simulink model "HCU_V2_Simulink"  (R2025b)
settings: Solver=FixedStepDiscrete  StartTime=0.0  StopTime=10.0  FixedStep=0.01  RelTol=1e-3
libraries: simulink x30, hdlsllib x9, etargetslib x7
(part 1 of 2)
settings Model: Creator=Yusha  LastModifiedBy=Yusha
settings OptimizationCC: DefaultParameterBehavior=Inlined  EnhancedBackFolding=on  PassReuseOutputArgsAs=Individual arguments  ZeroExternalMemoryAtStartup=off  ZeroInternalMemoryAtStartup=off  OptimizeBlockOrder=speed  DifferentSizesBufferReuse=on  OptimizationCustomize=off  EfficientTunableParamExpr=on
settings DebuggingCC: ParameterTunabilityLossMsg=error
settings HardwareCC: ProdBitPerPointer=32.0  ProdBitPerSizeT=32.0  ProdBitPerPtrDiffT=32.0  ProdLargestAtomicInteger=Long  ProdLargestAtomicFloat=Double  ProdWordSize=32.0  ProdHWDeviceType=ARM Compatible->ARM Cortex-M
settings SFSimCC: MATLABDynamicMemAlloc=off
settings RTWCC: SystemTargetFile=ert.tlc  GenCodeOnly=on  TemplateMakefile=ert_default_tmf  Description=Embedded Coder
settings CodeAppCC: ForceParamTrailComments=on  IgnoreCustomStorageClasses=off  OperatorAnnotations=on  SimulinkDataObjDesc=on  SFDataObjDesc=on  InsertBlockDesc=on
settings ERTTargetCC: ERTCustomFileTemplate=example_file_process.tlc  TargetLangStandard=C99 (ISO)

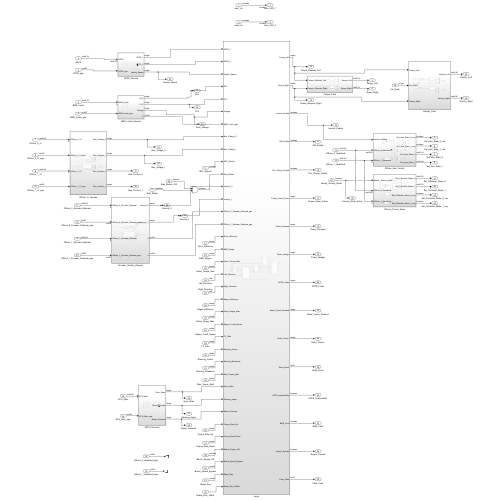
[thumbnail: Simulink's stored preview of the top-level diagram]
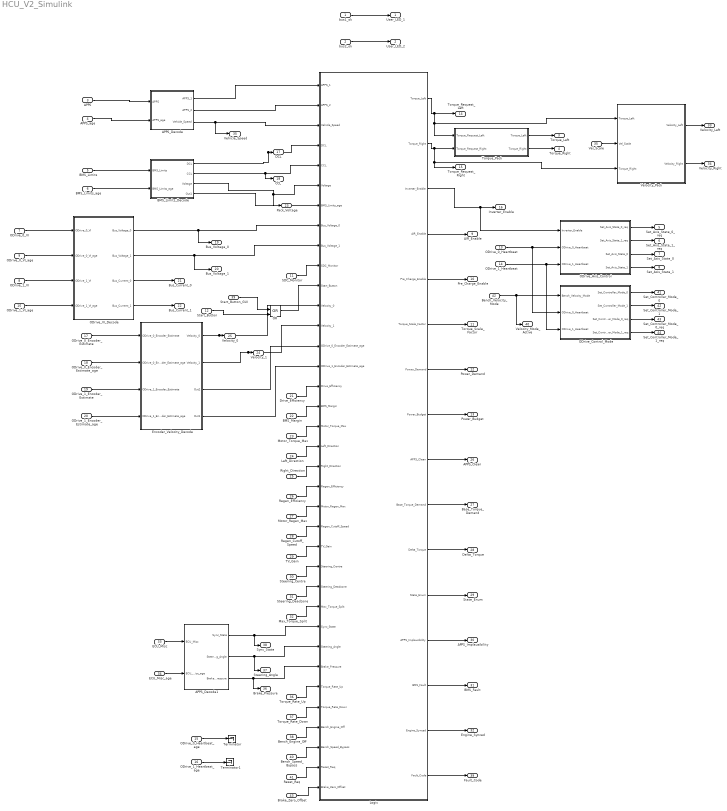
== system HCU_V2_Simulink ==
  bus1_ok : Inport  OutDataTypeStr=boolean
  bus2_ok : Inport  Port=2  OutDataTypeStr=boolean
  APPS : Inport  Port=3
  APPS_age : Inport  Port=4  OutDataTypeStr=uint32
  BMS_Limits : Inport  Port=5  OutDataTypeStr=uint8
  BMS_Limits_age : Inport  Port=6  OutDataTypeStr=uint32
  ODrive_0_VI : Inport  Port=7  OutDataTypeStr=uint8  PortDimensions=8
  ODrive_1_VI : Inport  Port=8  OutDataTypeStr=uint8  PortDimensions=8
  ODrive_0_VI_age : Inport  Port=9  OutDataTypeStr=uint32
  ODrive_1_VI_age : Inport  Port=10  OutDataTypeStr=uint32
  SDC_Monitor : Inport  Port=11  OutDataTypeStr=boolean
  Start_Button : Inport  Port=12  OutDataTypeStr=boolean
  ODrive_0_Heartbeat : Inport  Port=13  OutDataTypeStr=uint8  PortDimensions=8
  ODrive_1_Heartbeat : Inport  Port=14
  ODrive_0_Heartbeat_age : Inport  Port=15  OutDataTypeStr=uint32
  ODrive_1_Heartbeat_age : Inport  Port=16  OutDataTypeStr=uint32
  ODrive_0_Encoder_Estimate : Inport  Port=17  OutDataTypeStr=uint8  PortDimensions=8
  ODrive_0_Encoder_Estimate_age : Inport  Port=18  OutDataTypeStr=uint32
  ODrive_1_Encoder_Estimate : Inport  Port=19  OutDataTypeStr=uint8  PortDimensions=8
  ODrive_1_Encoder_Estimate_age : Inport  Port=20  OutDataTypeStr=uint32
  Drive_Efficiency : Inport  Port=21  OutDataTypeStr=single
  BMS_Margin : Inport  Port=22  OutDataTypeStr=single
  Motor_Torque_Max : Inport  Port=23  OutDataTypeStr=single
  Left_Direction : Inport  Port=24  OutDataTypeStr=int8
  Right_Direction : Inport  Port=25  OutDataTypeStr=int8
  Regen_Efficiency : Inport  Port=26  OutDataTypeStr=single
  Motor_Regen_Max : Inport  Port=27  OutDataTypeStr=single
  Regen_Cutoff_Speed : Inport  Port=28  OutDataTypeStr=single
  TV_Gain : Inport  Port=29
  Steering_Centre : Inport  Port=30
  Steering_Deadzone : Inport  Port=31
  Max_Torque_Split : Inport  Port=32
  ECU_Misc : Inport  Port=33  OutDataTypeStr=uint8  PortDimensions=8
  ECU_Misc_age : Inport  Port=34  OutDataTypeStr=uint32
  Vel_Scale : Inport  Port=35  OutDataTypeStr=single
  Torque_Rate_Up : Inport  Port=36
  Torque_Rate_Down : Inport  Port=37
  Bench_Engine_Off : Inport  Port=38  OutDataTypeStr=boolean
  Start_Button_GUI : Inport  Port=39
  Bench_Speed_Bypass : Inport  Port=40
  Reset_Req : Inport  Port=41
  Bench_Velocity_Mode : Inport  Port=42  OutDataTypeStr=boolean
  Brake_Zero_Offset : Inport  Port=43
  APPS_Decode : Subsystem
  APPS_Decode1 : Subsystem
  BMS_Limits_Decode : Subsystem
  Encoder_Velocity_Decode : Subsystem
  Logic : Subsystem
  ODrive_Axis_Control : Subsystem
  ODrive_Control_Mode : Subsystem
  ODrive_VI_Decode : Subsystem
  OR : Logic  Operator=OR  IconShape=distinctive  AllPortsSameDT=off  OutDataTypeStr=boolean
  Terminator : Terminator
  Terminator1 : Terminator
  Torque_Pack : Subsystem
  Velocity_Pack : Subsystem
  User_LED_1 : Outport  OutDataTypeStr=boolean
  User_LED_2 : Outport  Port=2  OutDataTypeStr=boolean
  Torque_Left : Outport  Port=3
  Torque_Right : Outport  Port=4
  Set_Axis_State_0_req : Outport  Port=5
  Set_Axis_State_1_req : Outport  Port=6
  Set_Axis_State_0 : Outport  Port=7
  Set_Axis_State_1 : Outport  Port=8
  AIR_Enable : Outport  Port=9
  Pre_Charge_Enable : Outport  Port=10
  Torque_Scale_Factor : Outport  Port=11
  Power_Demand : Outport  Port=12
  Power_Budget : Outport  Port=13
  Torque_Request_Left : Outport  Port=14
  Torque_Request_Right : Outport  Port=15
  Inverter_Enable : Outport  Port=16
  DCL : Outport  Port=17
  CCL : Outport  Port=18
  Bus_Voltage_0 : Outport  Port=19
  Bus_Voltage_1 : Outport  Port=20
  Bus_Current_0 : Outport  Port=21
  Bus_Current_1 : Outport  Port=22
  Pack_Voltage : Outport  Port=23
  Velocity_1 : Outport  Port=24
  Velocity_0 : Outport  Port=25
  APPS_Clean : Outport  Port=26
  Base_Torque_Demand : Outport  Port=27
  "Delta_Torque " : Outport  Port=28
  State_Enum : Outport  Port=29
  APPS_Implausibility : Outport  Port=30
  BMS_Fault : Outport  Port=31
  Engine_Synced : Outport  Port=32
  Velocity_Left : Outport  Port=33
  Velocity_Right : Outport  Port=34
  Vehicle_Speed : Outport  Port=35
  Brake_Pressure : Outport  Port=36
  Steering_Angle : Outport  Port=37
  Sync_State : Outport  Port=38
  Fault_Code : Outport  Port=39
  Velocity_Mode_Active : Outport  Port=40
  Set_Controller_Mode_0 : Outport  Port=41
  Set_Controller_Mode_1 : Outport  Port=42
  Set_Controller_Mode_0_req : Outport  Port=43
  Set_Controller_Mode_1_req : Outport  Port=44
  wires:
  bus2_ok/1 -> User_LED_2/1
  bus1_ok/1 -> User_LED_1/1
  APPS/1 -> APPS_Decode/1(APPS)
  APPS_age/1 -> APPS_Decode/2(APPS_age)
  APPS_Decode/1(APPS_1) -> Logic/1(APPS_1)
  APPS_Decode/2(APPS_2) -> Logic/2(APPS_2)
  BMS_Limits/1 -> BMS_Limits_Decode/1(BMS_Limits)
  BMS_Limits_age/1 -> BMS_Limits_Decode/2(BMS_Limits_age)
  BMS_Limits_Decode/1(DCL) -> DCL/1, Logic/4(DCL)
  BMS_Limits_Decode/2(CCL) -> CCL/1, Logic/5(CCL)
  BMS_Limits_Decode/3(Voltage) -> Pack_Voltage/1, Logic/6(Voltage)
  ODrive_0_VI/1 -> ODrive_VI_Decode/1(ODrive_0_VI)
  ODrive_0_VI_age/1 -> ODrive_VI_Decode/2(ODrive_0_VI_age)
  ODrive_1_VI/1 -> ODrive_VI_Decode/3(ODrive_1_VI)
  ODrive_1_VI_age/1 -> ODrive_VI_Decode/4(ODrive_1_VI_age)
  ODrive_VI_Decode/1(Bus_Voltage_0) -> Bus_Voltage_0/1, Logic/8(Bus_Voltage_0)
  ODrive_VI_Decode/2(Bus_Voltage_1) -> Bus_Voltage_1/1, Logic/9(Bus_Voltage_1)
  Logic/1(Torque_Left) -> Torque_Pack/1(Torque_Request_Left), Velocity_Pack/1(Torque_Left), Torque_Request_Left/1
  Logic/2(Torque_Right) -> Torque_Request_Right/1, Velocity_Pack/3(Torque_Right), Torque_Pack/2(Torque_Request_Right)
  Torque_Pack/1(Torque_Left) -> Torque_Left/1
  Torque_Pack/2(Torque_Right) -> Torque_Right/1
  Logic/3(Inverter_Enable) -> ODrive_Axis_Control/1(Inverter_Enable), Inverter_Enable/1
  ODrive_0_Heartbeat/1 -> ODrive_Axis_Control/2(ODrive_0_Heartbeat), ODrive_Control_Mode/2(ODrive_0_Heartbeat)
  ODrive_1_Heartbeat/1 -> ODrive_Control_Mode/3(ODrive_1_Heartbeat), ODrive_Axis_Control/3(ODrive_1_Heartbeat)
  ODrive_Axis_Control/1(Set_Axis_State_0_req) -> Set_Axis_State_0_req/1
  ODrive_Axis_Control/2(Set_Axis_State_1_req) -> Set_Axis_State_1_req/1
  ODrive_Axis_Control/3(Set_Axis_State_0) -> Set_Axis_State_0/1
  ODrive_Axis_Control/4(Set_Axis_State_1) -> Set_Axis_State_1/1
  Logic/4(AIR_Enable) -> AIR_Enable/1
  Logic/5(Pre_Charge_Enable) -> Pre_Charge_Enable/1
  ODrive_0_Heartbeat_age/1 -> Terminator/1
  ODrive_1_Heartbeat_age/1 -> Terminator1/1
  ODrive_0_Encoder_Estimate/1 -> Encoder_Velocity_Decode/1(ODrive_0_Encoder_Estimate)
  ODrive_0_Encoder_Estimate_age/1 -> Encoder_Velocity_Decode/2(ODrive_0_Encoder_Estimate_age)
  ODrive_1_Encoder_Estimate/1 -> Encoder_Velocity_Decode/3(ODrive_1_Encoder_Estimate)
  ODrive_1_Encoder_Estimate_age/1 -> Encoder_Velocity_Decode/4(ODrive_1_Encoder_Estimate_age)
  Encoder_Velocity_Decode/1(Velocity_0) -> Logic/12(Velocity_0), Velocity_0/1
  Encoder_Velocity_Decode/2(Velocity_1) -> Velocity_1/1, Logic/13(Velocity_1)
  Encoder_Velocity_Decode/3(Out2) -> Logic/14(ODrive_0_Encoder_Estimate_age)
  Encoder_Velocity_Decode/4(Out1) -> Logic/15(ODrive_1_Encoder_Estimate_age)
  BMS_Limits_Decode/4(Out1) -> Logic/7(BMS_Limits_age)
  Drive_Efficiency/1 -> Logic/16(Drive_Efficiency)
  BMS_Margin/1 -> Logic/17(BMS_Margin)
  Motor_Torque_Max/1 -> Logic/18(Motor_Torque_Max)
  Left_Direction/1 -> Logic/19(Left_Direction)
  Right_Direction/1 -> Logic/20(Right_Direction)
  Logic/6(Torque_Scale_Factor) -> Torque_Scale_Factor/1
  Logic/7(Power_Demand) -> Power_Demand/1
  Logic/8(Power_Budget) -> Power_Budget/1
  Regen_Efficiency/1 -> Logic/21(Regen_Efficiency)
  Motor_Regen_Max/1 -> Logic/22(Motor_Regen_Max)
  Regen_Cutoff_Speed/1 -> Logic/23(Regen_Cutoff_Speed)
  ODrive_VI_Decode/3(Bus_Current_0) -> Bus_Current_0/1
  ODrive_VI_Decode/4(Bus_Current_1) -> Bus_Current_1/1
  Logic/9(APPS_Clean) -> APPS_Clean/1
  Logic/10(Base_Torque_Demand) -> Base_Torque_Demand/1
  TV_Gain/1 -> Logic/24(TV_Gain)
  Steering_Centre/1 -> Logic/25(Steering_Centre)
  Steering_Deadzone/1 -> Logic/26(Steering_Deadzone)
  Max_Torque_Split/1 -> Logic/27(Max_Torque_Split)
  Logic/11("Delta_Torque ") -> "Delta_Torque "/1
  Logic/12(State_Enum) -> State_Enum/1
  Logic/13(APPS_Implausibility) -> APPS_Implausibility/1
  Logic/14(BMS_Fault) -> BMS_Fault/1
  ECU_Misc/1 -> APPS_Decode1/1(ECU_Misc)
  ECU_Misc_age/1 -> APPS_Decode1/2(ECU_Misc_age)
  APPS_Decode1/2(Steering_Angle) -> Steering_Angle/1, Logic/29(Steering_Angle)
  APPS_Decode1/3(Brake_Pressure) -> Brake_Pressure/1, Logic/30(Brake_Pressure)
  APPS_Decode1/1(Sync_State) -> Sync_State/1, Logic/28(Sync_State)
  Logic/15(Engine_Synced) -> Engine_Synced/1
  Vel_Scale/1 -> Velocity_Pack/2(Vel_Scale)
  Velocity_Pack/1(Velocity_Left) -> Velocity_Left/1
  Velocity_Pack/2(Velocity_Right) -> Velocity_Right/1
  Torque_Rate_Up/1 -> Logic/31(Torque_Rate_Up)
  Torque_Rate_Down/1 -> Logic/32(Torque_Rate_Down)
  Bench_Engine_Off/1 -> Logic/33(Bench_Engine_Off)
  OR/1 -> Logic/11(Start_Button)
  SDC_Monitor/1 -> Logic/10(SDC_Monitor)
  Start_Button_GUI/1 -> OR/1
  APPS_Decode/3(Vehicle_Speed) -> Vehicle_Speed/1, Logic/3(Vehicle_Speed)
  Bench_Speed_Bypass/1 -> Logic/34(Bench_Speed_Bypass)
  Start_Button/1 -> OR/2
  Logic/16(Fault_Code) -> Fault_Code/1
  Reset_Req/1 -> Logic/35(Reset_Req)
  Bench_Velocity_Mode/1 -> Velocity_Mode_Active/1, ODrive_Control_Mode/1(Bench_Velocity_Mode)
  ODrive_Control_Mode/1(Set_Controller_Mode_0) -> Set_Controller_Mode_0/1
  ODrive_Control_Mode/2(Set_Controller_Mode_1) -> Set_Controller_Mode_1/1
  ODrive_Control_Mode/3(Set_Controller_Mode_0_req) -> Set_Controller_Mode_0_req/1
  ODrive_Control_Mode/4(Set_Controller_Mode_1_req) -> Set_Controller_Mode_1_req/1
  Brake_Zero_Offset/1 -> Logic/36(Brake_Zero_Offset)

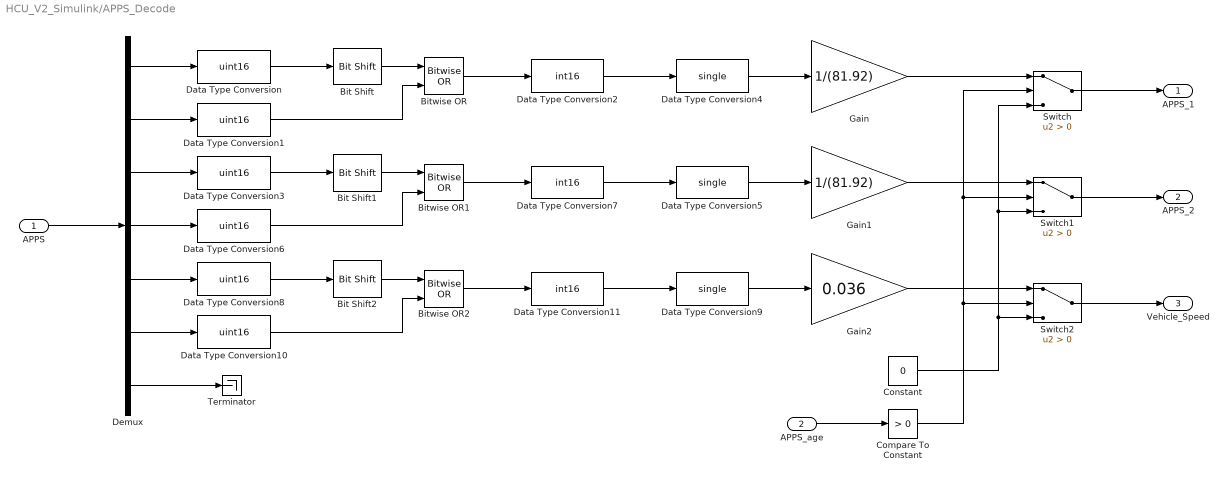
== system HCU_V2_Simulink/APPS_Decode ==
  APPS : Inport  OutDataTypeStr=uint8  PortDimensions=8
  APPS_age : Inport  Port=2
  Bit Shift : hdlsllib/Logic and Bit Operations/Bit Shift  mode=Shift Left Logical  N=8
  Bit Shift1 : hdlsllib/Logic and Bit Operations/Bit Shift  mode=Shift Left Logical  N=8
  Bit Shift2 : hdlsllib/Logic and Bit Operations/Bit Shift  mode=Shift Left Logical  N=8
  Bitwise OR : simulink/Logic and Bit Operations/Bitwise Operator  logicop=OR  UseBitMask=off  NumInputPorts=2  BitMask=bin2dec('11011001')  BitMaskRealWorld=Stored Integer
      settings: LibrarySourceBlock=|
      | simulink/Quick Insert/Logic and Bit
      | Operations/Bitwise OR
  Bitwise OR1 : simulink/Logic and Bit Operations/Bitwise Operator  logicop=OR  UseBitMask=off  NumInputPorts=2  BitMask=bin2dec('11011001')  BitMaskRealWorld=Stored Integer
      settings: LibrarySourceBlock=|
      | simulink/Quick Insert/Logic and Bit
      | Operations/Bitwise OR
  Bitwise OR2 : simulink/Logic and Bit Operations/Bitwise Operator  logicop=OR  UseBitMask=off  NumInputPorts=2  BitMask=bin2dec('11011001')  BitMaskRealWorld=Stored Integer
      settings: LibrarySourceBlock=|
      | simulink/Quick Insert/Logic and Bit
      | Operations/Bitwise OR
  Compare To Constant : simulink/Logic and Bit Operations/Compare To Constant  relop=>  const=0  OutDataTypeStr=boolean
  Constant : Constant  Value=0  OutDataTypeStr=single
  Data Type Conversion{,1,3,6,8,10} (6 alike) : DataTypeConversion  OutDataTypeStr=uint16  SaturateOnIntegerOverflow=off  RndMeth=Floor
  Data Type Conversion11 : DataTypeConversion  OutDataTypeStr=int16  ConvertRealWorld=Stored Integer (SI)  SaturateOnIntegerOverflow=off  RndMeth=Floor
  Data Type Conversion2 : DataTypeConversion  OutDataTypeStr=int16  ConvertRealWorld=Stored Integer (SI)  SaturateOnIntegerOverflow=off  RndMeth=Floor
  Data Type Conversion4 : DataTypeConversion  OutDataTypeStr=single  SaturateOnIntegerOverflow=off  RndMeth=Floor
  Data Type Conversion5 : DataTypeConversion  OutDataTypeStr=single  SaturateOnIntegerOverflow=off  RndMeth=Floor
  Data Type Conversion7 : DataTypeConversion  OutDataTypeStr=int16  ConvertRealWorld=Stored Integer (SI)  SaturateOnIntegerOverflow=off  RndMeth=Floor
  Data Type Conversion9 : DataTypeConversion  OutDataTypeStr=single  SaturateOnIntegerOverflow=off  RndMeth=Floor
  Demux : Demux  Outputs=[1 1 1 1 1 1 2]
  Gain : Gain  Gain=1/(81.92)
  Gain1 : Gain  Gain=1/(81.92)
  Gain2 : Gain  Gain=0.036
  Switch : Switch  Criteria=u2 > Threshold  SaturateOnIntegerOverflow=off  InputSameDT=off
  Switch1 : Switch  Criteria=u2 > Threshold  SaturateOnIntegerOverflow=off  InputSameDT=off
  Switch2 : Switch  Criteria=u2 > Threshold  SaturateOnIntegerOverflow=off  InputSameDT=off
  Terminator : Terminator
  APPS_1 : Outport
  APPS_2 : Outport  Port=2
  Vehicle_Speed : Outport  Port=3
  wires:
  Data Type Conversion5/1 -> Gain1/1
  Data Type Conversion4/1 -> Gain/1
  Demux/4 -> Data Type Conversion6/1
  Demux/2 -> Data Type Conversion1/1
  Data Type Conversion1/1 -> Bitwise OR/2
  Bit Shift1/1 -> Bitwise OR1/1
  Bit Shift/1 -> Bitwise OR/1
  Data Type Conversion3/1 -> Bit Shift1/1
  Data Type Conversion/1 -> Bit Shift/1
  Demux/3 -> Data Type Conversion3/1
  Data Type Conversion6/1 -> Bitwise OR1/2
  Bitwise OR/1 -> Data Type Conversion2/1
  Demux/1 -> Data Type Conversion/1
  Bitwise OR1/1 -> Data Type Conversion7/1
  APPS/1 -> Demux/1
  Data Type Conversion2/1 -> Data Type Conversion4/1
  Data Type Conversion7/1 -> Data Type Conversion5/1
  Gain/1 -> Switch/1
  Switch/1 -> APPS_1/1
  Gain1/1 -> Switch1/1
  Switch1/1 -> APPS_2/1
  APPS_age/1 -> Compare To Constant/1
  Compare To Constant/1 -> Switch2/2, Switch1/2, Switch/2
  Constant/1 -> Switch2/3, Switch1/3, Switch/3
  Demux/7 -> Terminator/1
  Demux/6 -> Data Type Conversion10/1
  Data Type Conversion11/1 -> Data Type Conversion9/1
  Data Type Conversion10/1 -> Bitwise OR2/2
  Bit Shift2/1 -> Bitwise OR2/1
  Bitwise OR2/1 -> Data Type Conversion11/1
  Data Type Conversion8/1 -> Bit Shift2/1
  Demux/5 -> Data Type Conversion8/1
  Data Type Conversion9/1 -> Gain2/1
  Gain2/1 -> Switch2/1
  Switch2/1 -> Vehicle_Speed/1

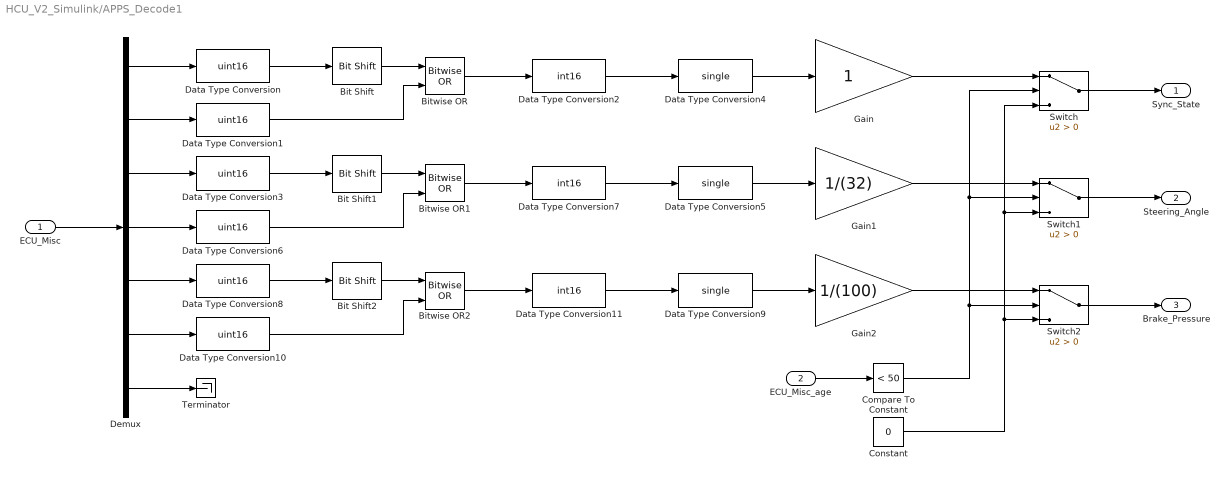
== system HCU_V2_Simulink/APPS_Decode1 ==
  ECU_Misc : Inport
  ECU_Misc_age : Inport  Port=2
  Bit Shift : hdlsllib/Logic and Bit Operations/Bit Shift  mode=Shift Left Logical  N=8
  Bit Shift1 : hdlsllib/Logic and Bit Operations/Bit Shift  mode=Shift Left Logical  N=8
  Bit Shift2 : hdlsllib/Logic and Bit Operations/Bit Shift  mode=Shift Left Logical  N=8
  Bitwise OR : simulink/Logic and Bit Operations/Bitwise Operator  logicop=OR  UseBitMask=off  NumInputPorts=2  BitMask=bin2dec('11011001')  BitMaskRealWorld=Stored Integer
      settings: LibrarySourceBlock=|
      | simulink/Quick Insert/Logic and Bit
      | Operations/Bitwise OR
  Bitwise OR1 : simulink/Logic and Bit Operations/Bitwise Operator  logicop=OR  UseBitMask=off  NumInputPorts=2  BitMask=bin2dec('11011001')  BitMaskRealWorld=Stored Integer
      settings: LibrarySourceBlock=|
      | simulink/Quick Insert/Logic and Bit
      | Operations/Bitwise OR
  Bitwise OR2 : simulink/Logic and Bit Operations/Bitwise Operator  logicop=OR  UseBitMask=off  NumInputPorts=2  BitMask=bin2dec('11011001')  BitMaskRealWorld=Stored Integer
      settings: LibrarySourceBlock=|
      | simulink/Quick Insert/Logic and Bit
      | Operations/Bitwise OR
  Compare To Constant : simulink/Logic and Bit Operations/Compare To Constant  relop=<  const=50  OutDataTypeStr=boolean
  Constant : Constant  Value=0  OutDataTypeStr=single
  Data Type Conversion{,1,3,6,8,10} (6 alike) : DataTypeConversion  OutDataTypeStr=uint16  SaturateOnIntegerOverflow=off  RndMeth=Floor
  Data Type Conversion11 : DataTypeConversion  OutDataTypeStr=int16  ConvertRealWorld=Stored Integer (SI)  SaturateOnIntegerOverflow=off  RndMeth=Floor
  Data Type Conversion2 : DataTypeConversion  OutDataTypeStr=int16  ConvertRealWorld=Stored Integer (SI)  SaturateOnIntegerOverflow=off  RndMeth=Floor
  Data Type Conversion4 : DataTypeConversion  OutDataTypeStr=single  SaturateOnIntegerOverflow=off  RndMeth=Floor
  Data Type Conversion5 : DataTypeConversion  OutDataTypeStr=single  SaturateOnIntegerOverflow=off  RndMeth=Floor
  Data Type Conversion7 : DataTypeConversion  OutDataTypeStr=int16  ConvertRealWorld=Stored Integer (SI)  SaturateOnIntegerOverflow=off  RndMeth=Floor
  Data Type Conversion9 : DataTypeConversion  OutDataTypeStr=single  SaturateOnIntegerOverflow=off  RndMeth=Floor
  Demux : Demux  Outputs=[1 1 1 1 1 1 2]
  Gain : Gain
  Gain1 : Gain  Gain=1/(32)
  Gain2 : Gain  Gain=1/(100)
  Switch : Switch  Criteria=u2 > Threshold  SaturateOnIntegerOverflow=off  InputSameDT=off
  Switch1 : Switch  Criteria=u2 > Threshold  SaturateOnIntegerOverflow=off  InputSameDT=off
  Switch2 : Switch  Criteria=u2 > Threshold  SaturateOnIntegerOverflow=off  InputSameDT=off
  Terminator : Terminator
  Sync_State : Outport
  Steering_Angle : Outport  Port=2
  Brake_Pressure : Outport  Port=3
  wires:
  Data Type Conversion5/1 -> Gain1/1
  Data Type Conversion4/1 -> Gain/1
  Demux/4 -> Data Type Conversion6/1
  Demux/2 -> Data Type Conversion1/1
  Data Type Conversion1/1 -> Bitwise OR/2
  Bit Shift1/1 -> Bitwise OR1/1
  Bit Shift/1 -> Bitwise OR/1
  Data Type Conversion3/1 -> Bit Shift1/1
  Data Type Conversion/1 -> Bit Shift/1
  Demux/3 -> Data Type Conversion3/1
  Data Type Conversion6/1 -> Bitwise OR1/2
  Bitwise OR/1 -> Data Type Conversion2/1
  Demux/1 -> Data Type Conversion/1
  Bitwise OR1/1 -> Data Type Conversion7/1
  Data Type Conversion2/1 -> Data Type Conversion4/1
  Data Type Conversion7/1 -> Data Type Conversion5/1
  Gain/1 -> Switch/1
  Gain1/1 -> Switch1/1
  Compare To Constant/1 -> Switch2/2, Switch1/2, Switch/2
  Constant/1 -> Switch2/3, Switch1/3, Switch/3
  Demux/7 -> Terminator/1
  Bitwise OR2/1 -> Data Type Conversion11/1
  Data Type Conversion8/1 -> Bit Shift2/1
  Data Type Conversion11/1 -> Data Type Conversion9/1
  Data Type Conversion9/1 -> Gain2/1
  Data Type Conversion10/1 -> Bitwise OR2/2
  Bit Shift2/1 -> Bitwise OR2/1
  Demux/5 -> Data Type Conversion8/1
  Demux/6 -> Data Type Conversion10/1
  ECU_Misc/1 -> Demux/1
  ECU_Misc_age/1 -> Compare To Constant/1
  Gain2/1 -> Switch2/1
  Switch/1 -> Sync_State/1
  Switch1/1 -> Steering_Angle/1
  Switch2/1 -> Brake_Pressure/1

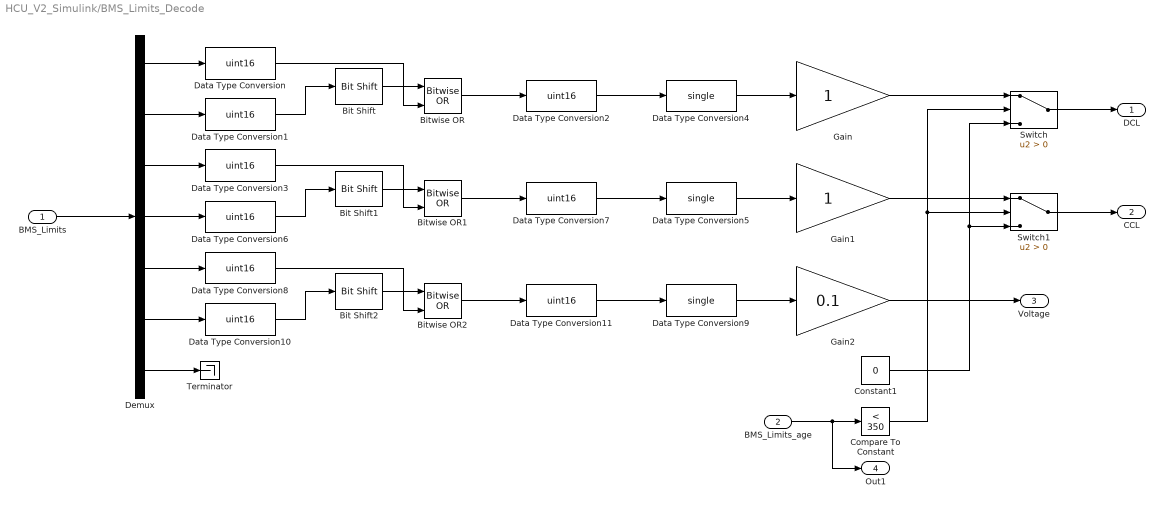
== system HCU_V2_Simulink/BMS_Limits_Decode ==
  BMS_Limits : Inport
  BMS_Limits_age : Inport  Port=2
  Bit Shift : hdlsllib/Logic and Bit Operations/Bit Shift  mode=Shift Left Logical  N=8
  Bit Shift1 : hdlsllib/Logic and Bit Operations/Bit Shift  mode=Shift Left Logical  N=8
  Bit Shift2 : hdlsllib/Logic and Bit Operations/Bit Shift  mode=Shift Left Logical  N=8
  Bitwise OR : simulink/Logic and Bit Operations/Bitwise Operator  logicop=OR  UseBitMask=off  NumInputPorts=2  BitMask=bin2dec('11011001')  BitMaskRealWorld=Stored Integer
      settings: LibrarySourceBlock=|
      | simulink/Quick Insert/Logic and Bit
      | Operations/Bitwise OR
  Bitwise OR1 : simulink/Logic and Bit Operations/Bitwise Operator  logicop=OR  UseBitMask=off  NumInputPorts=2  BitMask=bin2dec('11011001')  BitMaskRealWorld=Stored Integer
      settings: LibrarySourceBlock=|
      | simulink/Quick Insert/Logic and Bit
      | Operations/Bitwise OR
  Bitwise OR2 : simulink/Logic and Bit Operations/Bitwise Operator  logicop=OR  UseBitMask=off  NumInputPorts=2  BitMask=bin2dec('11011001')  BitMaskRealWorld=Stored Integer
      settings: LibrarySourceBlock=|
      | simulink/Quick Insert/Logic and Bit
      | Operations/Bitwise OR
  Compare To Constant : simulink/Logic and Bit Operations/Compare To Constant  relop=<  const=350  OutDataTypeStr=boolean
  Constant1 : Constant  Value=0  OutDataTypeStr=single
  Data Type Conversion{,1,3,6,8,10} (6 alike) : DataTypeConversion  OutDataTypeStr=uint16  SaturateOnIntegerOverflow=off  RndMeth=Floor
  Data Type Conversion11 : DataTypeConversion  OutDataTypeStr=uint16  ConvertRealWorld=Stored Integer (SI)  SaturateOnIntegerOverflow=off  RndMeth=Floor
  Data Type Conversion2 : DataTypeConversion  OutDataTypeStr=uint16  ConvertRealWorld=Stored Integer (SI)  SaturateOnIntegerOverflow=off  RndMeth=Floor
  Data Type Conversion4 : DataTypeConversion  OutDataTypeStr=single  SaturateOnIntegerOverflow=off  RndMeth=Floor
  Data Type Conversion5 : DataTypeConversion  OutDataTypeStr=single  SaturateOnIntegerOverflow=off  RndMeth=Floor
  Data Type Conversion7 : DataTypeConversion  OutDataTypeStr=uint16  ConvertRealWorld=Stored Integer (SI)  SaturateOnIntegerOverflow=off  RndMeth=Floor
  Data Type Conversion9 : DataTypeConversion  OutDataTypeStr=single  SaturateOnIntegerOverflow=off  RndMeth=Floor
  Demux : Demux  Outputs=[1 1 1 1 1 1 2]
  Gain : Gain
  Gain1 : Gain
  Gain2 : Gain  Gain=0.1
  Switch : Switch  Criteria=u2 > Threshold  SaturateOnIntegerOverflow=off  InputSameDT=off
  Switch1 : Switch  Criteria=u2 > Threshold  SaturateOnIntegerOverflow=off  InputSameDT=off
  Terminator : Terminator
  DCL : Outport
  CCL : Outport  Port=2
  Voltage : Outport  Port=3
  Out1 : Outport  Port=4
  wires:
  Data Type Conversion5/1 -> Gain1/1
  Data Type Conversion4/1 -> Gain/1
  Demux/4 -> Data Type Conversion6/1
  Demux/2 -> Data Type Conversion1/1
  Demux/3 -> Data Type Conversion3/1
  Bitwise OR/1 -> Data Type Conversion2/1
  Demux/1 -> Data Type Conversion/1
  Bitwise OR1/1 -> Data Type Conversion7/1
  BMS_Limits/1 -> Demux/1
  Data Type Conversion2/1 -> Data Type Conversion4/1
  Data Type Conversion7/1 -> Data Type Conversion5/1
  Gain/1 -> Switch/1
  Gain1/1 -> Switch1/1
  Compare To Constant/1 -> Switch1/2, Switch/2
  Data Type Conversion1/1 -> Bit Shift/1
  Bit Shift/1 -> Bitwise OR/1
  Data Type Conversion/1 -> Bitwise OR/2
  Data Type Conversion6/1 -> Bit Shift1/1
  Bit Shift1/1 -> Bitwise OR1/1
  Data Type Conversion3/1 -> Bitwise OR1/2
  Data Type Conversion11/1 -> Data Type Conversion9/1
  Gain2/1 -> Voltage/1
  Data Type Conversion9/1 -> Gain2/1
  Constant1/1 -> Switch/3, Switch1/3
  BMS_Limits_age/1 -> Out1/1, Compare To Constant/1
  Switch/1 -> DCL/1
  Switch1/1 -> CCL/1
  Demux/7 -> Terminator/1
  Data Type Conversion8/1 -> Bitwise OR2/2
  Data Type Conversion10/1 -> Bit Shift2/1
  Bitwise OR2/1 -> Data Type Conversion11/1
  Bit Shift2/1 -> Bitwise OR2/1
  Demux/6 -> Data Type Conversion10/1
  Demux/5 -> Data Type Conversion8/1

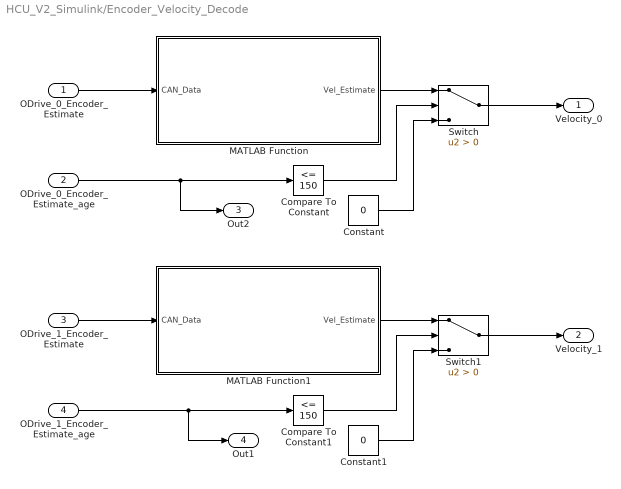
== system HCU_V2_Simulink/Encoder_Velocity_Decode ==
  ODrive_0_Encoder_Estimate : Inport  PortDimensions=8
  ODrive_0_Encoder_Estimate_age : Inport  Port=2  OutDataTypeStr=uint32
  ODrive_1_Encoder_Estimate : Inport  Port=3
  ODrive_1_Encoder_Estimate_age : Inport  Port=4  OutDataTypeStr=uint32
  Compare To Constant : simulink/Logic and Bit Operations/Compare To Constant  relop=<=  const=150  OutDataTypeStr=boolean
  Compare To Constant1 : simulink/Logic and Bit Operations/Compare To Constant  relop=<=  const=150  OutDataTypeStr=boolean
  Constant : Constant  Value=0  OutDataTypeStr=single
  Constant1 : Constant  Value=0  OutDataTypeStr=single
  MATLAB Function : MATLAB Function  TreatAsAtomicUnit=on
  MATLAB Function1 : MATLAB Function  TreatAsAtomicUnit=on
  Switch : Switch  Criteria=u2 > Threshold  SaturateOnIntegerOverflow=off  InputSameDT=off
  Switch1 : Switch  Criteria=u2 > Threshold  SaturateOnIntegerOverflow=off  InputSameDT=off
  Velocity_0 : Outport
  Velocity_1 : Outport  Port=2
  Out2 : Outport  Port=3
  Out1 : Outport  Port=4
  wires:
  MATLAB Function1/1(Vel_Estimate) -> Switch1/1
  ODrive_0_Encoder_Estimate_age/1 -> Out2/1, Compare To Constant/1
  MATLAB Function/1(Vel_Estimate) -> Switch/1
  ODrive_0_Encoder_Estimate/1 -> MATLAB Function/1(CAN_Data)
  ODrive_1_Encoder_Estimate_age/1 -> Out1/1, Compare To Constant1/1
  Compare To Constant/1 -> Switch/2
  ODrive_1_Encoder_Estimate/1 -> MATLAB Function1/1(CAN_Data)
  Constant/1 -> Switch/3
  Compare To Constant1/1 -> Switch1/2
  Constant1/1 -> Switch1/3
  Switch/1 -> Velocity_0/1
  Switch1/1 -> Velocity_1/1

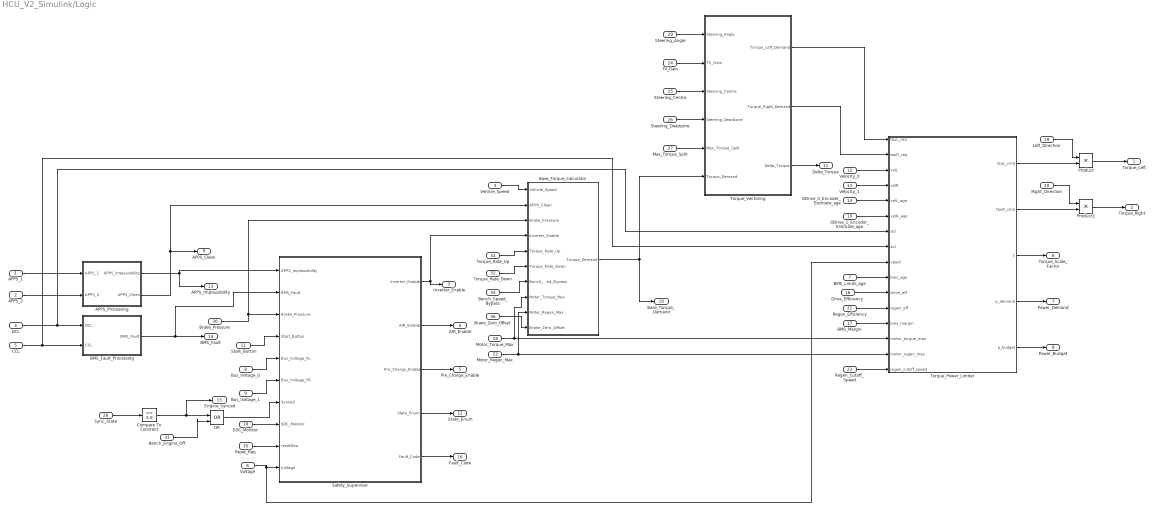
== system HCU_V2_Simulink/Logic ==
  APPS_1 : Inport
  APPS_2 : Inport  Port=2
  Vehicle_Speed : Inport  Port=3
  DCL : Inport  Port=4
  CCL : Inport  Port=5
  Voltage : Inport  Port=6
  BMS_Limits_age : Inport  Port=7
  Bus_Voltage_0 : Inport  Port=8
  Bus_Voltage_1 : Inport  Port=9
  SDC_Monitor : Inport  Port=10
  Start_Button : Inport  Port=11
  Velocity_0 : Inport  Port=12
  Velocity_1 : Inport  Port=13
  ODrive_0_Encoder_Estimate_age : Inport  Port=14
  ODrive_1_Encoder_Estimate_age : Inport  Port=15
  Drive_Efficiency : Inport  Port=16
  BMS_Margin : Inport  Port=17
  Motor_Torque_Max : Inport  Port=18
  Left_Direction : Inport  Port=19
  Right_Direction : Inport  Port=20
  Regen_Efficiency : Inport  Port=21
  Motor_Regen_Max : Inport  Port=22
  Regen_Cutoff_Speed : Inport  Port=23
  TV_Gain : Inport  Port=24
  Steering_Centre : Inport  Port=25
  Steering_Deadzone : Inport  Port=26
  Max_Torque_Split : Inport  Port=27
  Sync_State : Inport  Port=28
  Steering_Angle : Inport  Port=29
  Brake_Pressure : Inport  Port=30
  Torque_Rate_Up : Inport  Port=31
  Torque_Rate_Down : Inport  Port=32
  Bench_Engine_Off : Inport  Port=33
  Bench_Speed_Bypass : Inport  Port=34
  Reset_Req : Inport  Port=35
  Brake_Zero_Offset : Inport  Port=36
  APPS_Processing : Subsystem
  BMS_Fault_Processing : Subsystem
  Base_Torque_Calculator : Subsystem
  Compare To Constant : simulink/Logic and Bit Operations/Compare To Constant  relop===  const=3.0  OutDataTypeStr=boolean
  OR : Logic  Operator=OR  IconShape=distinctive  AllPortsSameDT=off  OutDataTypeStr=boolean
  Product : Product
  Product1 : Product
  Safety_Supervisor : Stateflow chart  TreatAsAtomicUnit=on
      settings: PortSchema="{\"entries\":[{\"content\":{\"sides\":[{\"content\":{\"connectorIds\":[\"In2\",\"In3\",\"In5\",\"In6\",\"In7\",\"In8\",\"In4\",\"In9\",\"In10\",\"In1\"]},\"type\":\"ConnectorPlacement.EquallySpacedRectSide\",\"uuid\":\"a4faffcb-836f-46f5-904b-8ae12aac25e8\"},{\"content\":{\"connectorIds\":[\"Out2\",\"Out1\",\"Out3\",\"Out4\",\"Out5\"],\"side\":\"RIGHT\"},\"type\":\"ConnectorPlacement.EquallySpacedRectSide\",\"uuid\":\"0660a6fe-5cdc-4355-a2c8-63e3455bf19c\"},{\"content\":{\"side\":\"TOP\"},\"type\":\"ConnectorPlacement.EquallySpacedRectSide\",\"uuid\":\"85cf7eed-5053-4a88-bcbe-9be750ede2ce\"}]},\"type\":\"ConnectorPlacement.EquallySpacedConnector\",\"uuid\":\"8a495802-9c76-4eed-af71-7fab7efc7756\"}],\"packageUris\":[\"http://schema.mathworks.com/mf0/Connector/R2020b\"],\"version\":\"1.0\"}"
  Torque_Power_Limiter : MATLAB Function  TreatAsAtomicUnit=on
  Torque_Vectoring : Subsystem
  Torque_Left : Outport
  Torque_Right : Outport  Port=2
  Inverter_Enable : Outport  Port=3
  AIR_Enable : Outport  Port=4
  Pre_Charge_Enable : Outport  Port=5
  Torque_Scale_Factor : Outport  Port=6
  Power_Demand : Outport  Port=7
  Power_Budget : Outport  Port=8
  APPS_Clean : Outport  Port=9
  Base_Torque_Demand : Outport  Port=10
  "Delta_Torque " : Outport  Port=11
  State_Enum : Outport  Port=12
  APPS_Implausibility : Outport  Port=13
  BMS_Fault : Outport  Port=14
  Engine_Synced : Outport  Port=15
  Fault_Code : Outport  Port=16
  wires:
  APPS_1/1 -> APPS_Processing/1(APPS_1)
  APPS_2/1 -> APPS_Processing/2(APPS_2)
  APPS_Processing/1(APPS_Implausibility) -> APPS_Implausibility/1, Safety_Supervisor/2(APPS_Implausibility)
  APPS_Processing/2(APPS_Clean) -> APPS_Clean/1, Base_Torque_Calculator/2(APPS_Clean)
  DCL/1 -> Torque_Power_Limiter/7(dcl), BMS_Fault_Processing/1(DCL)
  CCL/1 -> Torque_Power_Limiter/8(acl), BMS_Fault_Processing/2(CCL)
  Voltage/1 -> Torque_Power_Limiter/9(vpack), Safety_Supervisor/1(Voltage)
  Bus_Voltage_0/1 -> Safety_Supervisor/7(Bus_Voltage_FL)
  Bus_Voltage_1/1 -> Safety_Supervisor/8(Bus_Voltage_FR)
  SDC_Monitor/1 -> Safety_Supervisor/9(SDC_Monitor)
  Start_Button/1 -> Safety_Supervisor/6(Start_Button)
  Product/1 -> Torque_Left/1
  Product1/1 -> Torque_Right/1
  Brake_Pressure/1 -> Base_Torque_Calculator/3(Brake_Pressure), Safety_Supervisor/5(Brake_Pressure)
  Safety_Supervisor/1(AIR_Enable) -> AIR_Enable/1
  Safety_Supervisor/3(Pre_Charge_Enable) -> Pre_Charge_Enable/1
  Velocity_1/1 -> Torque_Power_Limiter/4(velR)
  Velocity_0/1 -> Torque_Power_Limiter/3(velL)
  ODrive_0_Encoder_Estimate_age/1 -> Torque_Power_Limiter/5(velL_age)
  ODrive_1_Encoder_Estimate_age/1 -> Torque_Power_Limiter/6(velR_age)
  Drive_Efficiency/1 -> Torque_Power_Limiter/11(drive_eff)
  BMS_Margin/1 -> Torque_Power_Limiter/13(bms_margin)
  Motor_Torque_Max/1 -> Base_Torque_Calculator/8(Motor_Torque_Max), Torque_Power_Limiter/14(motor_torque_max)
  Torque_Power_Limiter/1(tauL_cmd) -> Product/2
  Torque_Power_Limiter/2(tauR_cmd) -> Product1/2
  Right_Direction/1 -> Product1/1
  Left_Direction/1 -> Product/1
  Torque_Power_Limiter/3(s) -> Torque_Scale_Factor/1
  Torque_Power_Limiter/4(p_demand) -> Power_Demand/1
  Torque_Power_Limiter/5(p_budget) -> Power_Budget/1
  BMS_Limits_age/1 -> Torque_Power_Limiter/10(bms_age)
  Regen_Efficiency/1 -> Torque_Power_Limiter/12(regen_eff)
  Regen_Cutoff_Speed/1 -> Torque_Power_Limiter/16(regen_cutoff_speed)
  Base_Torque_Calculator/1(Torque_Demand) -> Torque_Vectoring/6(Torque_Demand), Base_Torque_Demand/1
  Safety_Supervisor/2(Inverter_Enable) -> Inverter_Enable/1, Base_Torque_Calculator/4(Inverter_Enable)
  Motor_Regen_Max/1 -> Base_Torque_Calculator/9(Motor_Regen_Max), Torque_Power_Limiter/15(motor_regen_max)
  Steering_Angle/1 -> Torque_Vectoring/1(Steering_Angle)
  TV_Gain/1 -> Torque_Vectoring/2(TV_Gain)
  Steering_Centre/1 -> Torque_Vectoring/3(Steering_Centre)
  Steering_Deadzone/1 -> Torque_Vectoring/4(Steering_Deadzone)
  Max_Torque_Split/1 -> Torque_Vectoring/5(Max_Torque_Split)
  Torque_Vectoring/3(Delta_Torque) -> "Delta_Torque "/1
  Torque_Vectoring/2(Torque_Right_Demand) -> Torque_Power_Limiter/2(tauR_req)
  Torque_Vectoring/1(Torque_Left_Demand) -> Torque_Power_Limiter/1(tauL_req)
  Safety_Supervisor/4(State_Enum) -> State_Enum/1
  BMS_Fault_Processing/1(BMS_Fault) -> BMS_Fault/1, Safety_Supervisor/3(BMS_Fault)
  Sync_State/1 -> Compare To Constant/1
  Torque_Rate_Up/1 -> Base_Torque_Calculator/5(Torque_Rate_Up)
  Torque_Rate_Down/1 -> Base_Torque_Calculator/6(Torque_Rate_Down)
  Compare To Constant/1 -> Engine_Synced/1, OR/1
  OR/1 -> Safety_Supervisor/4(Synced)
  Bench_Engine_Off/1 -> OR/2
  Vehicle_Speed/1 -> Base_Torque_Calculator/1(Vehicle_Speed)
  Bench_Speed_Bypass/1 -> Base_Torque_Calculator/7(Bench_Speed_Bypass)
  Safety_Supervisor/5(Fault_Code) -> Fault_Code/1
  Reset_Req/1 -> Safety_Supervisor/10(resetReq)
  Brake_Zero_Offset/1 -> Base_Torque_Calculator/10(Brake_Zero_Offset)

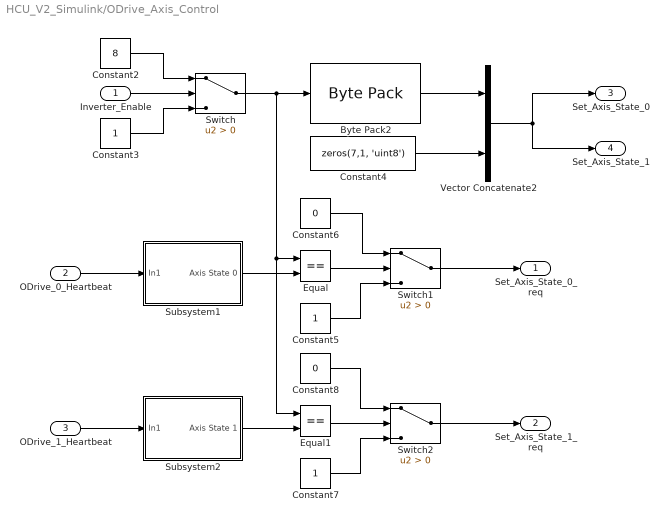
== system HCU_V2_Simulink/ODrive_Axis_Control ==
  Inverter_Enable : Inport
  ODrive_0_Heartbeat : Inport  Port=2  OutDataTypeStr=uint8  PortDimensions=8
  ODrive_1_Heartbeat : Inport  Port=3
  Byte Pack2 : etargetslib/Byte Pack  datatypes={'uint8'}  byteAlign=1
  Constant2 : Constant  Value=8  OutDataTypeStr=uint8
  Constant3 : Constant  OutDataTypeStr=uint8
  Constant4 : Constant  Value=zeros(7,1, 'uint8')  OutDataTypeStr=uint8
  Constant5 : Constant  OutDataTypeStr=boolean
  Constant6 : Constant  Value=0  OutDataTypeStr=boolean
  Constant7 : Constant  OutDataTypeStr=boolean
  Constant8 : Constant  Value=0  OutDataTypeStr=boolean
  Equal : RelationalOperator  Operator===  OutDataTypeStr=boolean  RndMeth=Simplest  InputSameDT=off
  Equal1 : RelationalOperator  Operator===  OutDataTypeStr=boolean  RndMeth=Simplest  InputSameDT=off
  Subsystem1 : Subsystem
  Subsystem2 : Subsystem
  Switch : Switch  Criteria=u2 > Threshold  SaturateOnIntegerOverflow=off  InputSameDT=off
  Switch1 : Switch  Criteria=u2 > Threshold  SaturateOnIntegerOverflow=off  InputSameDT=off
  Switch2 : Switch  Criteria=u2 > Threshold  SaturateOnIntegerOverflow=off  InputSameDT=off
  Vector Concatenate2 : Concatenate
  Set_Axis_State_0_req : Outport
  Set_Axis_State_1_req : Outport  Port=2
  Set_Axis_State_0 : Outport  Port=3
  Set_Axis_State_1 : Outport  Port=4
  wires:
  Switch2/1 -> Set_Axis_State_1_req/1
  Byte Pack2/1 -> Vector Concatenate2/1
  Vector Concatenate2/1 -> Set_Axis_State_1/1, Set_Axis_State_0/1
  Constant5/1 -> Switch1/3
  Constant8/1 -> Switch2/1
  Subsystem1/1(Axis State 0) -> Equal/2
  Switch/1 -> Equal1/1, Equal/1, Byte Pack2/1
  Subsystem2/1(Axis State 1) -> Equal1/2
  Constant7/1 -> Switch2/3
  Equal1/1 -> Switch2/2
  Switch1/1 -> Set_Axis_State_0_req/1
  ODrive_1_Heartbeat/1 -> Subsystem2/1(In1)
  Constant3/1 -> Switch/3
  Inverter_Enable/1 -> Switch/2
  ODrive_0_Heartbeat/1 -> Subsystem1/1(In1)
  Constant6/1 -> Switch1/1
  Constant2/1 -> Switch/1
  Equal/1 -> Switch1/2
  Constant4/1 -> Vector Concatenate2/2

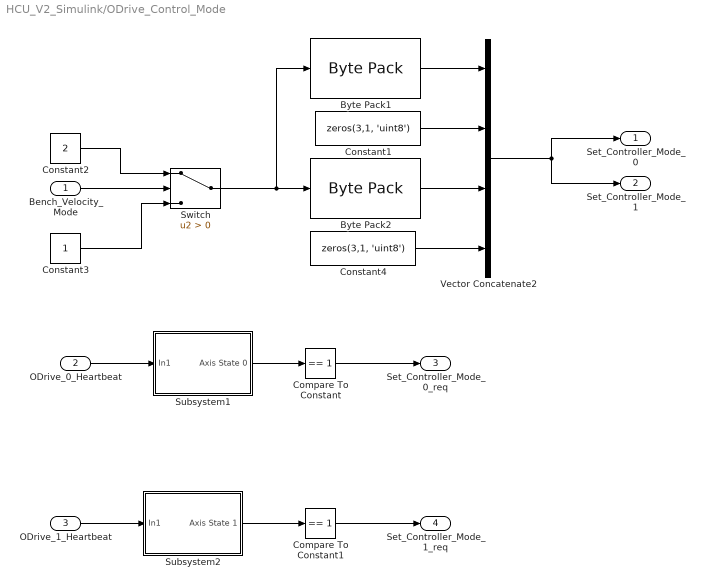
== system HCU_V2_Simulink/ODrive_Control_Mode ==
  Bench_Velocity_Mode : Inport
  ODrive_0_Heartbeat : Inport  Port=2  OutDataTypeStr=uint8  PortDimensions=8
  ODrive_1_Heartbeat : Inport  Port=3
  Byte Pack1 : etargetslib/Byte Pack  datatypes={'uint8'}  byteAlign=1
  Byte Pack2 : etargetslib/Byte Pack  datatypes={'uint8'}  byteAlign=1
  Compare To Constant : simulink/Logic and Bit Operations/Compare To Constant  relop===  const=1  OutDataTypeStr=boolean
  Compare To Constant1 : simulink/Logic and Bit Operations/Compare To Constant  relop===  const=1  OutDataTypeStr=boolean
  Constant1 : Constant  Value=zeros(3,1, 'uint8')  OutDataTypeStr=uint8
  Constant2 : Constant  Value=2  OutDataTypeStr=uint8
  Constant3 : Constant  OutDataTypeStr=uint8
  Constant4 : Constant  Value=zeros(3,1, 'uint8')  OutDataTypeStr=uint8
  Subsystem1 : Subsystem
  Subsystem2 : Subsystem
  Switch : Switch  Criteria=u2 > Threshold  SaturateOnIntegerOverflow=off  InputSameDT=off
  Vector Concatenate2 : Concatenate  NumInputs=4
  Set_Controller_Mode_0 : Outport
  Set_Controller_Mode_1 : Outport  Port=2
  Set_Controller_Mode_0_req : Outport  Port=3
  Set_Controller_Mode_1_req : Outport  Port=4
  wires:
  Switch/1 -> Byte Pack1/1, Byte Pack2/1
  ODrive_1_Heartbeat/1 -> Subsystem2/1(In1)
  Constant3/1 -> Switch/3
  Bench_Velocity_Mode/1 -> Switch/2
  ODrive_0_Heartbeat/1 -> Subsystem1/1(In1)
  Constant2/1 -> Switch/1
  Vector Concatenate2/1 -> Set_Controller_Mode_0/1, Set_Controller_Mode_1/1
  Byte Pack1/1 -> Vector Concatenate2/1
  Constant1/1 -> Vector Concatenate2/2
  Byte Pack2/1 -> Vector Concatenate2/3
  Constant4/1 -> Vector Concatenate2/4
  Subsystem1/1(Axis State 0) -> Compare To Constant/1
  Subsystem2/1(Axis State 1) -> Compare To Constant1/1
  Compare To Constant1/1 -> Set_Controller_Mode_1_req/1
  Compare To Constant/1 -> Set_Controller_Mode_0_req/1

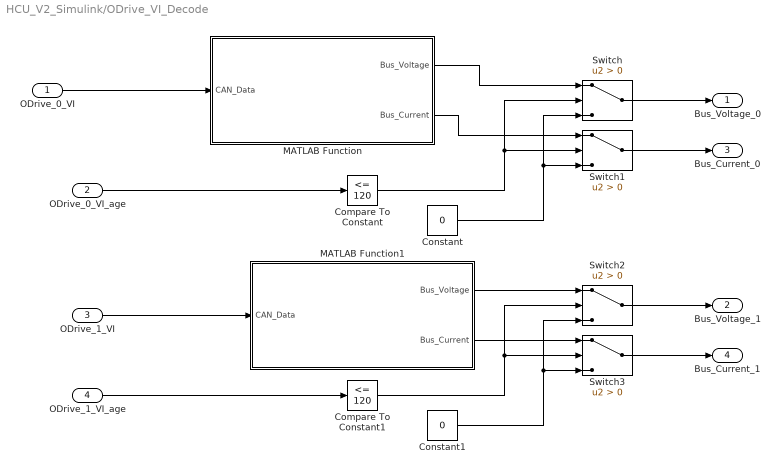
== system HCU_V2_Simulink/ODrive_VI_Decode ==
  ODrive_0_VI : Inport
  ODrive_0_VI_age : Inport  Port=2
  ODrive_1_VI : Inport  Port=3
  ODrive_1_VI_age : Inport  Port=4
  Compare To Constant : simulink/Logic and Bit Operations/Compare To Constant  relop=<=  const=120  OutDataTypeStr=boolean
  Compare To Constant1 : simulink/Logic and Bit Operations/Compare To Constant  relop=<=  const=120  OutDataTypeStr=boolean
  Constant : Constant  Value=0  OutDataTypeStr=single
  Constant1 : Constant  Value=0  OutDataTypeStr=single
  MATLAB Function : MATLAB Function  TreatAsAtomicUnit=on
  MATLAB Function1 : MATLAB Function  TreatAsAtomicUnit=on
  Switch{,1..3} (4 alike) : Switch  Criteria=u2 > Threshold  SaturateOnIntegerOverflow=off  InputSameDT=off
  Bus_Voltage_0 : Outport
  Bus_Voltage_1 : Outport  Port=2
  Bus_Current_0 : Outport  Port=3
  Bus_Current_1 : Outport  Port=4
  wires:
  Compare To Constant/1 -> Switch1/2, Switch/2
  Switch2/1 -> Bus_Voltage_1/1
  Switch1/1 -> Bus_Current_0/1
  Compare To Constant1/1 -> Switch3/2, Switch2/2
  Constant1/1 -> Switch2/3, Switch3/3
  MATLAB Function1/2(Bus_Current) -> Switch3/1
  ODrive_0_VI/1 -> MATLAB Function/1(CAN_Data)
  Switch/1 -> Bus_Voltage_0/1
  MATLAB Function/1(Bus_Voltage) -> Switch/1
  MATLAB Function1/1(Bus_Voltage) -> Switch2/1
  ODrive_0_VI_age/1 -> Compare To Constant/1
  MATLAB Function/2(Bus_Current) -> Switch1/1
  Switch3/1 -> Bus_Current_1/1
  Constant/1 -> Switch/3, Switch1/3
  ODrive_1_VI/1 -> MATLAB Function1/1(CAN_Data)
  ODrive_1_VI_age/1 -> Compare To Constant1/1

== system HCU_V2_Simulink/Torque_Pack ==
  Torque_Request_Left : Inport
  Torque_Request_Right : Inport  Port=2
  Byte Pack : etargetslib/Byte Pack  datatypes={'single'}  byteAlign=1
  Byte Pack1 : etargetslib/Byte Pack  datatypes={'single'}  byteAlign=1
  Constant : Constant  Value=zeros(4,1, 'uint8')  OutDataTypeStr=uint8
  Constant1 : Constant  Value=zeros(4,1, 'uint8')  OutDataTypeStr=uint8
  Vector Concatenate : Concatenate
  Vector Concatenate1 : Concatenate
  Torque_Left : Outport
  Torque_Right : Outport  Port=2
  wires:
  Torque_Request_Left/1 -> Byte Pack1/1
  Byte Pack/1 -> Vector Concatenate1/1
  Byte Pack1/1 -> Vector Concatenate/1
  Vector Concatenate/1 -> Torque_Left/1
  Constant1/1 -> Vector Concatenate1/2
  Constant/1 -> Vector Concatenate/2
  Vector Concatenate1/1 -> Torque_Right/1
  Torque_Request_Right/1 -> Byte Pack/1

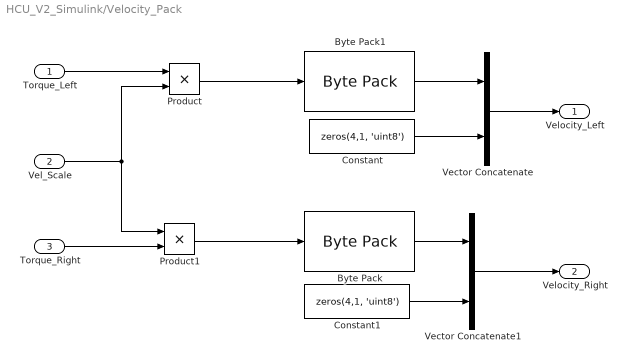
== system HCU_V2_Simulink/Velocity_Pack ==
  Torque_Left : Inport
  Vel_Scale : Inport  Port=2
  Torque_Right : Inport  Port=3
  Byte Pack : etargetslib/Byte Pack  datatypes={'single'}  byteAlign=1
  Byte Pack1 : etargetslib/Byte Pack  datatypes={'single'}  byteAlign=1
  Constant : Constant  Value=zeros(4,1, 'uint8')  OutDataTypeStr=uint8
  Constant1 : Constant  Value=zeros(4,1, 'uint8')  OutDataTypeStr=uint8
  Product : Product
  Product1 : Product
  Vector Concatenate : Concatenate
  Vector Concatenate1 : Concatenate
  Velocity_Left : Outport
  Velocity_Right : Outport  Port=2
  wires:
  Constant1/1 -> Vector Concatenate1/2
  Byte Pack/1 -> Vector Concatenate1/1
  Byte Pack1/1 -> Vector Concatenate/1
  Constant/1 -> Vector Concatenate/2
  Vector Concatenate/1 -> Velocity_Left/1
  Vector Concatenate1/1 -> Velocity_Right/1
  Torque_Left/1 -> Product/1
  Product/1 -> Byte Pack1/1
  Vel_Scale/1 -> Product/2, Product1/1
  Torque_Right/1 -> Product1/2
  Product1/1 -> Byte Pack/1

== system HCU_V2_Simulink/Logic/APPS_Processing ==
  APPS_1 : Inport
  APPS_2 : Inport  Port=2
  Abs : Abs  SaturateOnIntegerOverflow=off
  Compare To Constant : simulink/Logic and Bit Operations/Compare To Constant  relop=>  const=10  OutDataTypeStr=boolean
  Min : MinMax  Inputs=2
  Subtract : Sum  Inputs=+-
  APPS_Implausibility : Outport
  APPS_Clean : Outport  Port=2
  wires:
  APPS_2/1 -> Subtract/2, Min/2
  Min/1 -> APPS_Clean/1
  APPS_1/1 -> Subtract/1, Min/1
  Compare To Constant/1 -> APPS_Implausibility/1
  Abs/1 -> Compare To Constant/1
  Subtract/1 -> Abs/1

== system HCU_V2_Simulink/Logic/BMS_Fault_Processing ==
  DCL : Inport
  CCL : Inport  Port=2
  AND : Logic  IconShape=distinctive  AllPortsSameDT=off  OutDataTypeStr=boolean
  Compare To Constant : simulink/Logic and Bit Operations/Compare To Constant  relop===  const=0  OutDataTypeStr=boolean
  Compare To Constant1 : simulink/Logic and Bit Operations/Compare To Constant  relop===  const=0  OutDataTypeStr=boolean
  BMS_Fault : Outport
  wires:
  Compare To Constant/1 -> AND/1
  AND/1 -> BMS_Fault/1
  Compare To Constant1/1 -> AND/2
  DCL/1 -> Compare To Constant/1
  CCL/1 -> Compare To Constant1/1

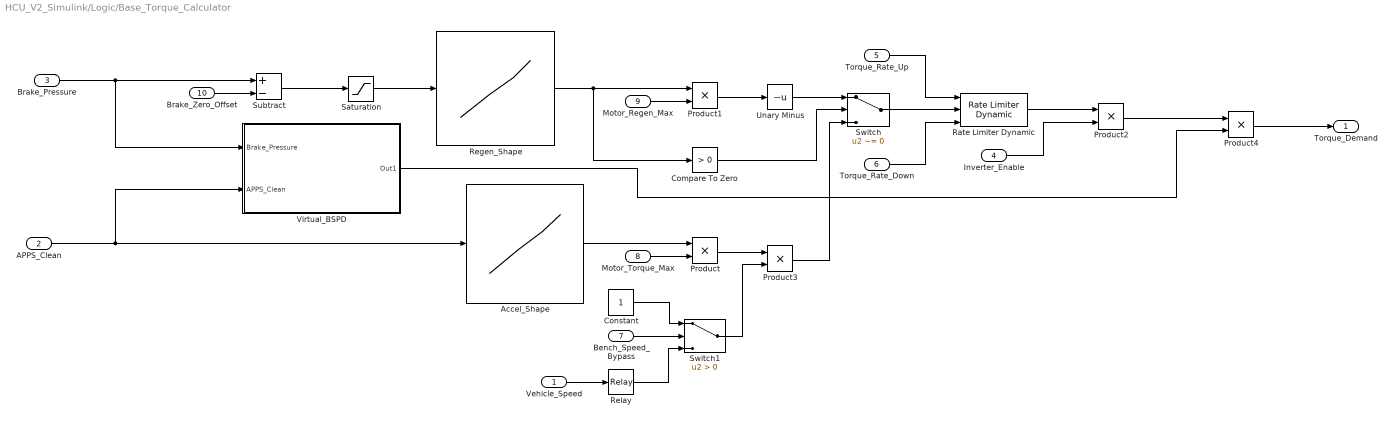
== system HCU_V2_Simulink/Logic/Base_Torque_Calculator ==
  Vehicle_Speed : Inport
  APPS_Clean : Inport  Port=2
  Brake_Pressure : Inport  Port=3
  Inverter_Enable : Inport  Port=4
  Torque_Rate_Up : Inport  Port=5
  Torque_Rate_Down : Inport  Port=6
  Bench_Speed_Bypass : Inport  Port=7
  Motor_Torque_Max : Inport  Port=8
  Motor_Regen_Max : Inport  Port=9
  Brake_Zero_Offset : Inport  Port=10
  Accel_Shape : Lookup_n-D  NumberOfTableDimensions=1  BreakpointsForDimension1=[0 3 10 25 50 75 100]  Table=[0 0 0.08 0.25 0.55 0.80 1.0]  ExtrapMethod=Clip  InternalRulePriority=Speed  RndMeth=Simplest
  Compare To Zero : simulink/Logic and Bit Operations/Compare To Zero  relop=>  OutDataTypeStr=boolean
  Constant : Constant  OutDataTypeStr=single
  Product{,1..4} (5 alike) : Product
  Rate Limiter Dynamic : simulink/Discontinuities/Rate Limiter Dynamic
  Regen_Shape : Lookup_n-D  NumberOfTableDimensions=1  BreakpointsForDimension1=[0 2 5 20 40 60]  Table=[0 0 0.2 0.6 0.9 1.0]  ExtrapMethod=Clip  InternalRulePriority=Speed  RndMeth=Simplest
  Relay : Relay  OnSwitchValue=5  OffSwitchValue=3
  Saturation : Saturate  UpperLimit=60  LowerLimit=0
  Subtract : Sum  Inputs=+-
  Switch : Switch  Criteria=u2 ~= 0  SaturateOnIntegerOverflow=off  InputSameDT=off
  Switch1 : Switch  Criteria=u2 > Threshold  SaturateOnIntegerOverflow=off  InputSameDT=off
  Unary Minus : UnaryMinus
  Virtual_BSPD : Subsystem
  Torque_Demand : Outport
  wires:
  APPS_Clean/1 -> Virtual_BSPD/2(APPS_Clean), Accel_Shape/1
  Accel_Shape/1 -> Product/1
  Motor_Torque_Max/1 -> Product/2
  Brake_Pressure/1 -> Virtual_BSPD/1(Brake_Pressure), Subtract/1
  Regen_Shape/1 -> Compare To Zero/1, Product1/1
  Motor_Regen_Max/1 -> Product1/2
  Product1/1 -> Unary Minus/1
  Unary Minus/1 -> Switch/1
  Compare To Zero/1 -> Switch/2
  Inverter_Enable/1 -> Product2/2
  Switch/1 -> Rate Limiter Dynamic/2
  Rate Limiter Dynamic/1 -> Product2/1
  Torque_Rate_Up/1 -> Rate Limiter Dynamic/1
  Torque_Rate_Down/1 -> Rate Limiter Dynamic/3
  Vehicle_Speed/1 -> Relay/1
  Product/1 -> Product3/1
  Product3/1 -> Switch/3
  Product2/1 -> Product4/1
  Product4/1 -> Torque_Demand/1
  Virtual_BSPD/1(Out1) -> Product4/2
  Bench_Speed_Bypass/1 -> Switch1/2
  Switch1/1 -> Product3/2
  Relay/1 -> Switch1/3
  Constant/1 -> Switch1/1
  Brake_Zero_Offset/1 -> Subtract/2
  Subtract/1 -> Saturation/1
  Saturation/1 -> Regen_Shape/1

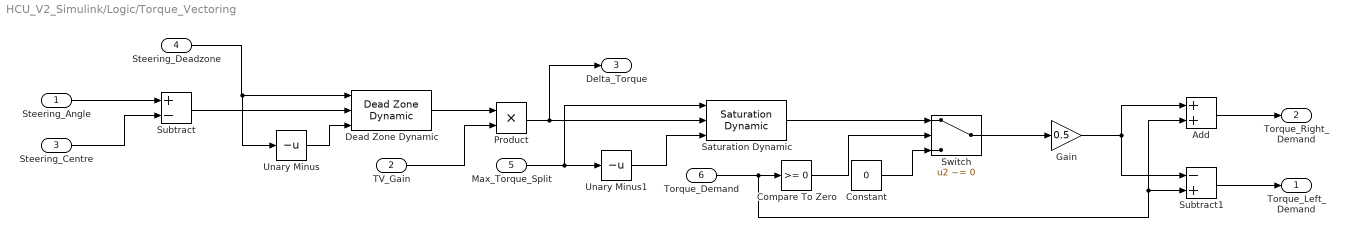
== system HCU_V2_Simulink/Logic/Torque_Vectoring ==
  Steering_Angle : Inport
  TV_Gain : Inport  Port=2
  Steering_Centre : Inport  Port=3
  Steering_Deadzone : Inport  Port=4
  Max_Torque_Split : Inport  Port=5
  Torque_Demand : Inport  Port=6
  Add : Sum  OutDataTypeStr=single
  Compare To Zero : simulink/Logic and Bit Operations/Compare To Zero  relop=>=  OutDataTypeStr=boolean
  Constant : Constant  Value=0  OutDataTypeStr=single
  Dead Zone Dynamic : simulink/Discontinuities/Dead Zone Dynamic
  Gain : Gain  Gain=0.5
  Product : Product
  Saturation Dynamic : simulink/Discontinuities/Saturation Dynamic  OutMin=[]  OutMax=[]  OutDataTypeStr=Inherit: Same as second input  OutDataType=fixdt(1, 16)  OutScaling=2^-10  DoSatur=off
  Subtract : Sum  Inputs=+-
  Subtract1 : Sum  Inputs=-+  OutDataTypeStr=single
  Switch : Switch  Criteria=u2 ~= 0  SaturateOnIntegerOverflow=off  InputSameDT=off
  Unary Minus : UnaryMinus
  Unary Minus1 : UnaryMinus
  Torque_Left_Demand : Outport
  Torque_Right_Demand : Outport  Port=2
  Delta_Torque : Outport  Port=3
  wires:
  Steering_Angle/1 -> Subtract/1
  Steering_Centre/1 -> Subtract/2
  Subtract/1 -> Dead Zone Dynamic/2
  Steering_Deadzone/1 -> Unary Minus/1, Dead Zone Dynamic/1
  Unary Minus/1 -> Dead Zone Dynamic/3
  Dead Zone Dynamic/1 -> Product/1
  TV_Gain/1 -> Product/2
  Product/1 -> Saturation Dynamic/2, Delta_Torque/1
  Max_Torque_Split/1 -> Unary Minus1/1, Saturation Dynamic/1
  Unary Minus1/1 -> Saturation Dynamic/3
  Torque_Demand/1 -> Compare To Zero/1, Add/2, Subtract1/2
  Saturation Dynamic/1 -> Switch/1
  Constant/1 -> Switch/3
  Switch/1 -> Gain/1
  Gain/1 -> Subtract1/1, Add/1
  Subtract1/1 -> Torque_Left_Demand/1
  Add/1 -> Torque_Right_Demand/1
  Compare To Zero/1 -> Switch/2

== system HCU_V2_Simulink/ODrive_Axis_Control/Subsystem1 ==
  In1 : Inport
  Data Type Conversion : DataTypeConversion  OutDataTypeStr=uint8  SaturateOnIntegerOverflow=off  RndMeth=Floor
  Demux : Demux  Outputs=[4 1 3]
  Terminator : Terminator
  Terminator1 : Terminator
  Axis State 0 : Outport
  wires:
  Demux/3 -> Terminator1/1
  Demux/1 -> Terminator/1
  Data Type Conversion/1 -> Axis State 0/1
  Demux/2 -> Data Type Conversion/1
  In1/1 -> Demux/1

== system HCU_V2_Simulink/ODrive_Axis_Control/Subsystem2 ==
  In1 : Inport
  Data Type Conversion : DataTypeConversion  OutDataTypeStr=uint8  SaturateOnIntegerOverflow=off  RndMeth=Floor
  Demux : Demux  Outputs=[4 1 3]
  Terminator : Terminator
  Terminator1 : Terminator
  Axis State 1 : Outport
  wires:
  Demux/3 -> Terminator1/1
  Demux/1 -> Terminator/1
  Data Type Conversion/1 -> Axis State 1/1
  Demux/2 -> Data Type Conversion/1
  In1/1 -> Demux/1

== system HCU_V2_Simulink/ODrive_Control_Mode/Subsystem1 ==
  In1 : Inport
  Data Type Conversion : DataTypeConversion  OutDataTypeStr=uint8  SaturateOnIntegerOverflow=off  RndMeth=Floor
  Demux : Demux  Outputs=[4 1 3]
  Terminator : Terminator
  Terminator1 : Terminator
  Axis State 0 : Outport
  wires:
  Demux/3 -> Terminator1/1
  Demux/1 -> Terminator/1
  Data Type Conversion/1 -> Axis State 0/1
  Demux/2 -> Data Type Conversion/1
  In1/1 -> Demux/1

== system HCU_V2_Simulink/ODrive_Control_Mode/Subsystem2 ==
  In1 : Inport
  Data Type Conversion : DataTypeConversion  OutDataTypeStr=uint8  SaturateOnIntegerOverflow=off  RndMeth=Floor
  Demux : Demux  Outputs=[4 1 3]
  Terminator : Terminator
  Terminator1 : Terminator
  Axis State 1 : Outport
  wires:
  Demux/3 -> Terminator1/1
  Demux/1 -> Terminator/1
  Data Type Conversion/1 -> Axis State 1/1
  Demux/2 -> Data Type Conversion/1
  In1/1 -> Demux/1

== system HCU_V2_Simulink/Logic/Base_Torque_Calculator/Virtual_BSPD ==
  Brake_Pressure : Inport
  APPS_Clean : Inport  Port=2
  AND : Logic  IconShape=distinctive  AllPortsSameDT=off  OutDataTypeStr=boolean
  AND1 : Logic  IconShape=distinctive  AllPortsSameDT=off  OutDataTypeStr=boolean
  Compare To Constant : simulink/Logic and Bit Operations/Compare To Constant  relop=>=  const=25  OutDataTypeStr=boolean
  Compare To Constant1 : simulink/Logic and Bit Operations/Compare To Constant  relop=>=  const=20  OutDataTypeStr=boolean
  Compare To Constant2 : simulink/Logic and Bit Operations/Compare To Constant  relop=<=  const=5  OutDataTypeStr=boolean
  NOT1 : Logic  Operator=NOT  IconShape=distinctive  AllPortsSameDT=off  OutDataTypeStr=boolean
  NOT2 : Logic  Operator=NOT  IconShape=distinctive  AllPortsSameDT=off  OutDataTypeStr=boolean
  OR : Logic  Operator=OR  IconShape=distinctive  AllPortsSameDT=off  OutDataTypeStr=boolean
  Unit Delay : UnitDelay  SampleTime=-1  HasFrameUpgradeWarning=on
  Out1 : Outport
  wires:
  OR/1 -> Unit Delay/1, NOT2/1
  Compare To Constant/1 -> AND/1
  Unit Delay/1 -> AND1/2
  Compare To Constant1/1 -> AND/2
  AND/1 -> OR/1
  NOT1/1 -> AND1/1
  Compare To Constant2/1 -> NOT1/1
  APPS_Clean/1 -> Compare To Constant2/1, Compare To Constant1/1
  AND1/1 -> OR/2
  NOT2/1 -> Out1/1
  Brake_Pressure/1 -> Compare To Constant/1

== matlab function HCU_V2_Simulink/ODrive_VI_Decode/MATLAB Function1 ==
  data: CAN_Data input; Bus_Voltage output; Bus_Current output
function [Bus_Voltage, Bus_Current] = decode_vbus(CAN_Data)
    d = uint8(CAN_Data(:));    % 8x1 uint8, orientation-proof

    % little-endian: byte0 = LSB ... byte3 = MSB
    v = bitor(bitor(           uint32(d(1)),      bitshift(uint32(d(2)),  8)), bitor(bitshift(uint32(d(3)), 16),   bitshift(uint32(d(4)), 24)));
    c = bitor(bitor(           uint32(d(5)),      bitshift(uint32(d(6)),  8)), bitor(bitshift(uint32(d(7)), 16),   bitshift(uint32(d(8)), 24)));

    Bus_Voltage = typecast(v, 'single');   % scalar uint32 -> scalar single (1x1)
    Bus_Current = typecast(c, 'single');
end

== matlab function HCU_V2_Simulink/ODrive_VI_Decode/MATLAB Function ==
  data: CAN_Data input; Bus_Voltage output; Bus_Current output
function [Bus_Voltage, Bus_Current] = decode_vbus(CAN_Data)
    d = uint8(CAN_Data(:));    % 8x1 uint8, orientation-proof

    % little-endian: byte0 = LSB ... byte3 = MSB
    v = bitor(bitor(           uint32(d(1)),      bitshift(uint32(d(2)),  8)), bitor(bitshift(uint32(d(3)), 16),   bitshift(uint32(d(4)), 24)));
    c = bitor(bitor(           uint32(d(5)),      bitshift(uint32(d(6)),  8)), bitor(bitshift(uint32(d(7)), 16),   bitshift(uint32(d(8)), 24)));

    Bus_Voltage = typecast(v, 'single');   % scalar uint32 -> scalar single (1x1)
    Bus_Current = typecast(c, 'single');
end
